simulink model "momentum based estimator"  (R2022a)
settings: Solver=VariableStepAuto  StartTime=0.0  StopTime=30  RelTol=1e-3
values from neighbouring files (symbols this model uses):
  Ib = diag([1.2416 1.2416 2*1.2416])    [momentum based estimator.m]
  k11 = wn1    (= 80)    [momentum based estimator.m]
  k12 = wn2^2/k22    (= 57.1428571429)    [momentum based estimator.m]
  k13 = wn3^3/k33/k23    (= 35.8139534884)    [momentum based estimator.m]
  k14 = wn4^4/k24/k34/k44    (= 33.3333333333)    [momentum based estimator.m]
  k15 = wn5^5/k25/k35/k45/k55    (= 30.2941176471)    [momentum based estimator.m]
  k22 = 1.4*wn2    (= 112)    [momentum based estimator.m]
  k23 = 2.15*wn3^2/k33    (= 94.6)    [momentum based estimator.m]
  k24 = 2.7*wn4^3/k34/k44    (= 71.4705882353)    [momentum based estimator.m]
  k25 = 3.4*wn5^4/k35/k45/k55    (= 63.6727272727)    [momentum based estimator.m]
  k33 = 1.75*wn3    (= 134.75)    [momentum based estimator.m]
  k34 = 3.4*wn4^2/k44    (= 145.714285714)    [momentum based estimator.m]
  k35 = 5.5*wn5^3/k55/k45    (= 113.3)    [momentum based estimator.m]
  k44 = 2.1*wn4    (= 189)    [momentum based estimator.m]
  k45 = 5*wn5^2/k55    (= 183.928571429)    [momentum based estimator.m]
  k55 = 2.8*wn5    (= 288.4)    [momentum based estimator.m]
  mass = 1.1    [momentum based estimator.m]
undefined symbols (not defined in the file or in its folder): DiscIntNeverNeededParam
settings Model: Creator=ThinkPad  LastModifiedBy=ThinkPad

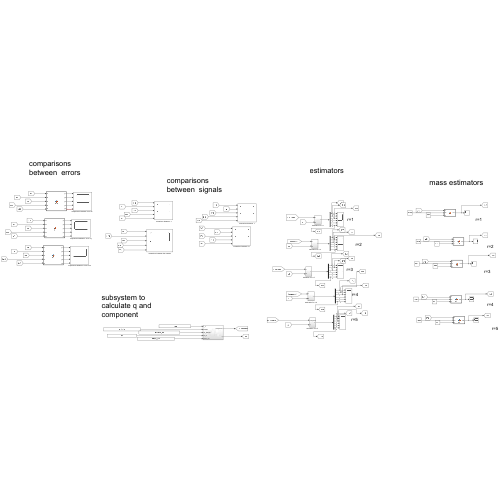
[thumbnail: Simulink's stored preview of the top-level diagram]
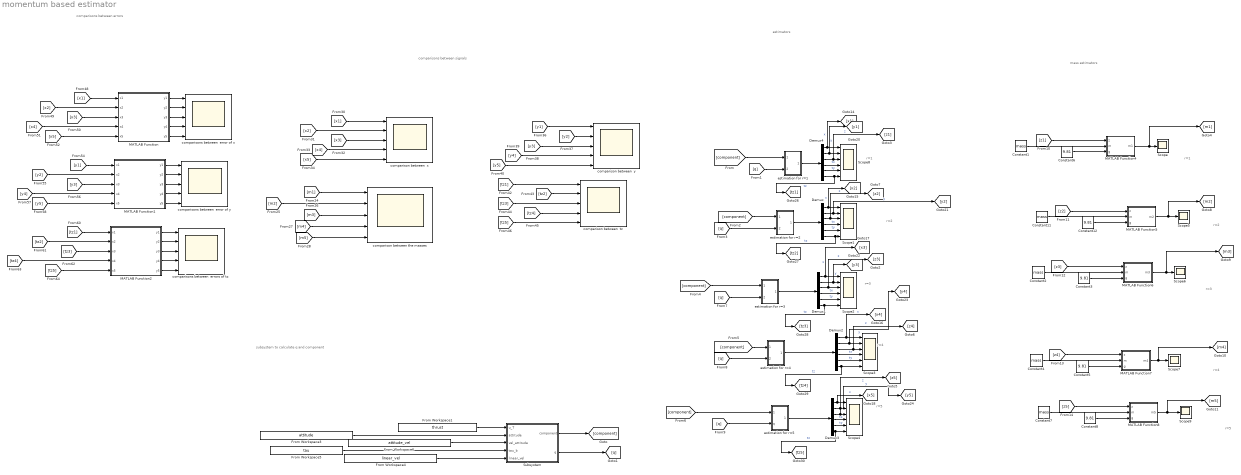
== system momentum based estimator ==
  note: r=1
  note: r=3
  note: r=2
  note: estimators
  note: comparisons between errors
  note: r=5
  note: r=4
  note: comparisons between signals
  note: mass estimators
  note: subsystem to calculate q and component
  note: r=1
  note: r=2
  note: r=3
  note: r=4
  note: r=5
  Constant{1..2,4,7,11} (5 alike) : Constant  Value=mass
  Constant{3,5..6,8,12} (5 alike) : Constant  Value=9.81
  Demux{,1..4} (5 alike) : Demux  Outputs=6
  From Workspace1 : FromWorkspace  VariableName=thrust  SampleTime=0.001
  From Workspace3 : FromWorkspace  VariableName=attitude  SampleTime=0.001
  From Workspace4 : FromWorkspace  VariableName=linear_vel  SampleTime=0.001
  From Workspace5 : FromWorkspace  VariableName=tau  SampleTime=0.001
  From Workspace6 : FromWorkspace  VariableName=attitude_vel  SampleTime=0.001
  MATLAB Function : MATLAB Function  TreatAsAtomicUnit=on
  MATLAB Function1 : MATLAB Function  TreatAsAtomicUnit=on
  MATLAB Function2 : MATLAB Function  TreatAsAtomicUnit=on
  MATLAB Function4 : MATLAB Function  TreatAsAtomicUnit=on
  MATLAB Function5 : MATLAB Function  TreatAsAtomicUnit=on
  MATLAB Function6 : MATLAB Function  TreatAsAtomicUnit=on
  MATLAB Function7 : MATLAB Function  TreatAsAtomicUnit=on
  MATLAB Function8 : MATLAB Function  TreatAsAtomicUnit=on
  Scope{,5..7,9} (5 alike) : Scope
  Scope{1..4,8} (5 alike) : Scope  NumInputPorts=6
  Subsystem : Subsystem
  comparison between  tz : Scope  NumInputPorts=5
  comparison between  x : Scope  NumInputPorts=5
  comparison between  y : Scope  NumInputPorts=5
  comparison between the masses : Scope  NumInputPorts=5
  comparisons between  error of x : Scope  NumInputPorts=5
  comparisons between  error of y : Scope  NumInputPorts=5
  comparisons between  errors of tz : Scope  NumInputPorts=5
  estimation for r=1 : Subsystem
  estimation for r=2 : Subsystem
  estimation for r=3 : Subsystem
  estimation for r=4 : Subsystem
  estimation for r=5 : Subsystem
  wires:
  Demux1/3 -> Scope2/3, [z3]  "z"
  [component] -> estimation for r=4/1(In1)
  Demux2/5 -> Scope3/5  "ty"
  [component] -> estimation for r=1/1(In1)
  Demux/3 -> [z2], Scope1/3  "z"
  estimation for r=2/1(Out1) -> Demux/1
  Demux/5 -> Scope1/5  "ty"
  [m5] -> comparison between the masses/5
  Demux4/6 -> [tz1], Scope8/6  "tz"
  Demux3/6 -> [tz5], Scope4/6  "tz"
  From Workspace3/1 -> Subsystem/2(attitude)
  Demux4/2 -> [y1], Scope8/2  "y"
  From Workspace6/1 -> Subsystem/3(vel_attitude)
  Demux4/3 -> [z1], Scope8/3  "z"
  estimation for r=5/1(Out1) -> Demux3/1
  Demux3/2 -> [y5], Scope4/2  "y"
  estimation for r=4/1(Out1) -> Demux2/1
  Demux/2 -> [y2], Scope1/2  "y"
  From Workspace5/1 -> Subsystem/4(tau_b)
  [x4] -> MATLAB Function/4(x4)
  [x2] -> MATLAB Function/2(x2)
  [q] -> estimation for r=4/2(In2)
  MATLAB Function1/5(y5) -> comparisons between  error of y/5
  [q] -> estimation for r=1/2(In2)
  [m2] -> comparison between the masses/2
  [y5] -> MATLAB Function1/5(x5)
  Subsystem/2(q) -> [q]
  MATLAB Function/2(y2) -> comparisons between  error of x/2
  [y2] -> MATLAB Function1/2(x2)
  [y1] -> MATLAB Function1/1(x1)
  [tz5] -> MATLAB Function2/5(x5)
  MATLAB Function2/5(y5) -> comparisons between  errors of tz/5
  MATLAB Function2/3(y3) -> comparisons between  errors of tz/3
  Demux2/3 -> [z4], Scope3/3  "z"
  From Workspace4/1 -> Subsystem/5(linear_vel)
  MATLAB Function1/3(y3) -> comparisons between  error of y/3
  Demux1/6 -> [tz3], Scope2/6  "tz"
  Demux3/4 -> Scope4/4  "tx"
  Demux2/4 -> Scope3/4  "tx"
  [component] -> estimation for r=3/1(In1)
  estimation for r=1/1(Out1) -> Demux4/1
  Demux3/1 -> [x5], Scope4/1  "x"
  MATLAB Function1/2(y2) -> comparisons between  error of y/2
  [component] -> estimation for r=5/1(component)
  Demux/1 -> [x2], Scope1/1  "x"
  From Workspace1/1 -> Subsystem/1(u_T)
  [tz3] -> comparison between  tz/3
  Demux2/6 -> [tz4], Scope3/6  "tz"
  [tz4] -> comparison between  tz/4
  [x1] -> comparison between  x/1
  Demux/6 -> [tz2], Scope1/6  "tz"
  Demux4/5 -> Scope8/5  "ty"
  Demux1/2 -> [y3], Scope2/2  "y"
  estimation for r=3/1(Out1) -> Demux1/1
  [tz1] -> comparison between  tz/1
  [q] -> estimation for r=5/2(q)
  [x5] -> comparison between  x/5
  [y4] -> comparison between  y/4
  [tz2] -> comparison between  tz/2
  [x4] -> comparison between  x/4
  [x3] -> comparison between  x/3
  [x2] -> comparison between  x/2
  [y1] -> comparison between  y/1
  [y3] -> comparison between  y/3
  [y2] -> comparison between  y/2
  [tz5] -> comparison between  tz/5
  [x3] -> MATLAB Function/3(x3)
  Demux3/3 -> [z5], Scope4/3  "z"
  [m4] -> comparison between the masses/4
  MATLAB Function/3(y3) -> comparisons between  error of x/3
  ? -> ?
  [y3] -> MATLAB Function1/3(x3)
  [y4] -> MATLAB Function1/4(x4)
  MATLAB Function/4(y4) -> comparisons between  error of x/4
  Demux2/2 -> [y4], Scope3/2  "y"
  Demux3/5 -> Scope4/5  "ty"
  [y5] -> comparison between  y/5
  [x5] -> MATLAB Function/5(x5)
  Demux1/5 -> Scope2/5  "ty"
  Demux2/1 -> [x4], Scope3/1  "x"
  [component] -> estimation for r=2/1(In1)
  [q] -> estimation for r=3/2(In2)
  Subsystem/1(component) -> [component]
  [x1] -> MATLAB Function/1(x1)
  Demux4/4 -> Scope8/4  "tx"
  Demux1/1 -> [x3], Scope2/1  "x"
  Demux4/1 -> [x1], Scope8/1  "x"
  [q] -> estimation for r=2/2(In2)
  Demux/4 -> Scope1/4  "tx"
  MATLAB Function/5(y5) -> comparisons between  error of x/5
  MATLAB Function/1(y1) -> comparisons between  error of x/1
  [tz2] -> MATLAB Function2/2(x2)
  Demux1/4 -> Scope2/4  "tx"
  MATLAB Function1/4(y4) -> comparisons between  error of y/4
  [m1] -> comparison between the masses/1
  MATLAB Function2/4(y4) -> comparisons between  errors of tz/4
  [tz4] -> MATLAB Function2/4(x4)
  [tz1] -> MATLAB Function2/1(x1)
  [tz3] -> MATLAB Function2/3(x3)
  MATLAB Function2/2(y2) -> comparisons between  errors of tz/2
  MATLAB Function2/1(y1) -> comparisons between  errors of tz/1
  [m3] -> comparison between the masses/3
  MATLAB Function1/1(y1) -> comparisons between  error of y/1
  [z1] -> MATLAB Function4/1(z)
  Constant1/1 -> MATLAB Function4/2(m)
  Constant6/1 -> MATLAB Function4/3(g)
  [z2] -> MATLAB Function5/1(z)
  Constant11/1 -> MATLAB Function5/2(m)
  Constant12/1 -> MATLAB Function5/3(g)
  MATLAB Function5/1(m2) -> Scope5/1, [m2]
  MATLAB Function6/1(m3) -> Scope6/1, [m3]
  Constant3/1 -> MATLAB Function6/3(g)
  Constant2/1 -> MATLAB Function6/2(m)
  [z3] -> MATLAB Function6/1(z)
  MATLAB Function7/1(m4) -> Scope7/1, [m4]
  Constant5/1 -> MATLAB Function7/3(g)
  Constant4/1 -> MATLAB Function7/2(m)
  [z4] -> MATLAB Function7/1(z)
  MATLAB Function8/1(m5) -> Scope9/1, [m5]
  Constant8/1 -> MATLAB Function8/3(g)
  Constant7/1 -> MATLAB Function8/2(m)
  [z5] -> MATLAB Function8/1(z)
  MATLAB Function4/1(m1) -> [m1], Scope/1

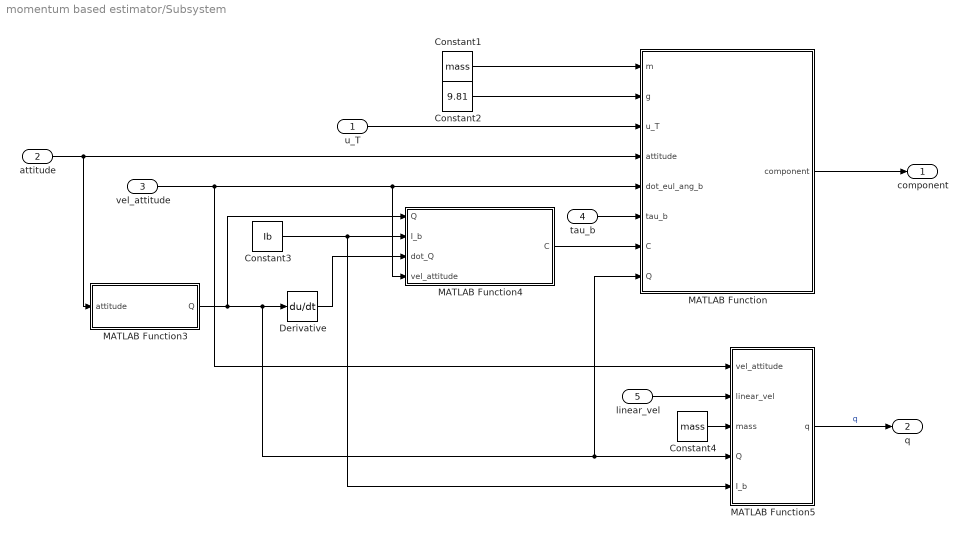
== system momentum based estimator/Subsystem ==
  u_T : Inport
  attitude : Inport  Port=2
  vel_attitude : Inport  Port=3
  tau_b : Inport  Port=4
  linear_vel : Inport  Port=5
  Constant1 : Constant  Value=mass
  Constant2 : Constant  Value=9.81
  Constant3 : Constant  Value=Ib
  Constant4 : Constant  Value=mass
  Derivative : Derivative
  MATLAB Function : MATLAB Function  TreatAsAtomicUnit=on
  MATLAB Function3 : MATLAB Function  TreatAsAtomicUnit=on
  MATLAB Function4 : MATLAB Function  TreatAsAtomicUnit=on
  MATLAB Function5 : MATLAB Function  TreatAsAtomicUnit=on
  component : Outport
  q : Outport  Port=2
  wires:
  Constant4/1 -> MATLAB Function5/3(mass)
  Constant1/1 -> MATLAB Function/1(m)
  MATLAB Function3/1(Q) -> Derivative/1, MATLAB Function5/4(Q), MATLAB Function/8(Q), MATLAB Function4/1(Q)
  Constant2/1 -> MATLAB Function/2(g)
  attitude/1 -> MATLAB Function3/1(attitude), MATLAB Function/4(attitude)
  Derivative/1 -> MATLAB Function4/3(dot_Q)
  Constant3/1 -> MATLAB Function5/5(I_b), MATLAB Function4/2(I_b)
  MATLAB Function4/1(C) -> MATLAB Function/7(C)
  MATLAB Function5/1(q) -> q/1  "q"
  tau_b/1 -> MATLAB Function/6(tau_b)
  u_T/1 -> MATLAB Function/3(u_T)
  MATLAB Function/1(component) -> component/1
  linear_vel/1 -> MATLAB Function5/2(linear_vel)
  vel_attitude/1 -> MATLAB Function5/1(vel_attitude), MATLAB Function4/4(vel_attitude), MATLAB Function/5(dot_eul_ang_b)

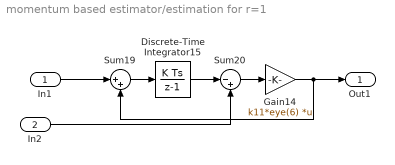
== system momentum based estimator/estimation for r=1 ==
  In1 : Inport
  In2 : Inport  Port=2
  Discrete-Time Integrator15 : DiscreteIntegrator  SampleTime=0.001  ICPrevOutput=DiscIntNeverNeededParam  ICPrevScaledInput=DiscIntNeverNeededParam
  Gain14 : Gain  Gain=k11*eye(6)  Multiplication=Matrix(K*u)
  Sum19 : Sum  Inputs=|++
  Sum20 : Sum  Inputs=|-+
  Out1 : Outport
  wires:
  Gain14/1 -> Out1/1, Sum19/2
  Sum20/1 -> Gain14/1
  In1/1 -> Sum19/1
  Discrete-Time Integrator15/1 -> Sum20/1
  Sum19/1 -> Discrete-Time Integrator15/1
  In2/1 -> Sum20/2

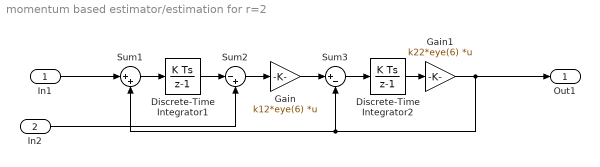
== system momentum based estimator/estimation for r=2 ==
  In1 : Inport
  In2 : Inport  Port=2
  Discrete-Time Integrator1 : DiscreteIntegrator  SampleTime=0.001  ICPrevOutput=DiscIntNeverNeededParam  ICPrevScaledInput=DiscIntNeverNeededParam
  Discrete-Time Integrator2 : DiscreteIntegrator  SampleTime=0.001  ICPrevOutput=DiscIntNeverNeededParam  ICPrevScaledInput=DiscIntNeverNeededParam
  Gain : Gain  Gain=k12*eye(6)  Multiplication=Matrix(K*u)
  Gain1 : Gain  Gain=k22*eye(6)  Multiplication=Matrix(K*u)
  Sum1 : Sum  Inputs=|++
  Sum2 : Sum  Inputs=|-+
  Sum3 : Sum  Inputs=|+-
  Out1 : Outport
  wires:
  Gain1/1 -> Out1/1, Sum1/2, Sum3/2
  Discrete-Time Integrator1/1 -> Sum2/1
  Sum2/1 -> Gain/1
  Sum3/1 -> Discrete-Time Integrator2/1
  Discrete-Time Integrator2/1 -> Gain1/1
  Gain/1 -> Sum3/1
  Sum1/1 -> Discrete-Time Integrator1/1
  In1/1 -> Sum1/1
  In2/1 -> Sum2/2

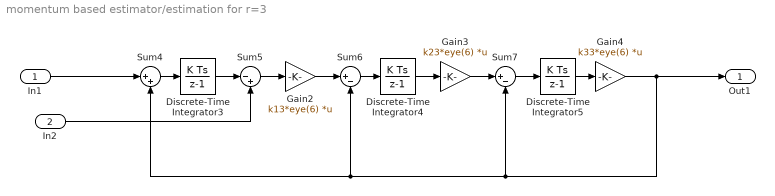
== system momentum based estimator/estimation for r=3 ==
  In1 : Inport
  In2 : Inport  Port=2
  Discrete-Time Integrator3 : DiscreteIntegrator  InitialCondition=0.001  SampleTime=-1  ICPrevOutput=DiscIntNeverNeededParam  ICPrevScaledInput=DiscIntNeverNeededParam
  Discrete-Time Integrator4 : DiscreteIntegrator  SampleTime=0.001  ICPrevOutput=DiscIntNeverNeededParam  ICPrevScaledInput=DiscIntNeverNeededParam
  Discrete-Time Integrator5 : DiscreteIntegrator  SampleTime=0.001  ICPrevOutput=DiscIntNeverNeededParam  ICPrevScaledInput=DiscIntNeverNeededParam
  Gain2 : Gain  Gain=k13*eye(6)  Multiplication=Matrix(K*u)
  Gain3 : Gain  Gain=k23*eye(6)  Multiplication=Matrix(K*u)
  Gain4 : Gain  Gain=k33*eye(6)  Multiplication=Matrix(K*u)
  Sum4 : Sum  Inputs=|++
  Sum5 : Sum  Inputs=|-+
  Sum6 : Sum  Inputs=|+-
  Sum7 : Sum  Inputs=|+-
  Out1 : Outport
  wires:
  Discrete-Time Integrator3/1 -> Sum5/1
  Sum6/1 -> Discrete-Time Integrator4/1
  Gain2/1 -> Sum6/1
  Sum7/1 -> Discrete-Time Integrator5/1
  Sum4/1 -> Discrete-Time Integrator3/1
  Discrete-Time Integrator5/1 -> Gain4/1
  Gain3/1 -> Sum7/1
  Discrete-Time Integrator4/1 -> Gain3/1
  Sum5/1 -> Gain2/1
  Gain4/1 -> Out1/1, Sum4/2, Sum6/2, Sum7/2
  In1/1 -> Sum4/1
  In2/1 -> Sum5/2

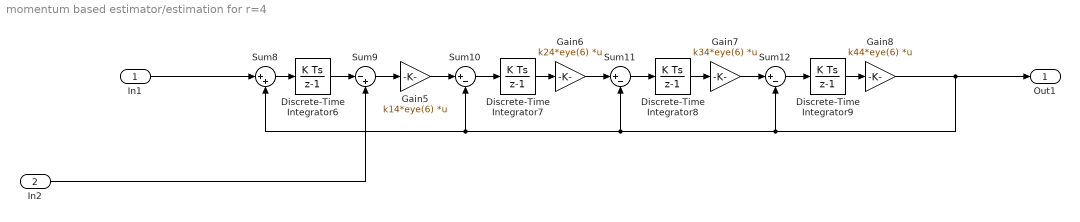
== system momentum based estimator/estimation for r=4 ==
  In1 : Inport
  In2 : Inport  Port=2
  Discrete-Time Integrator{6..9} (4 alike) : DiscreteIntegrator  SampleTime=0.001  ICPrevOutput=DiscIntNeverNeededParam  ICPrevScaledInput=DiscIntNeverNeededParam
  Gain5 : Gain  Gain=k14*eye(6)  Multiplication=Matrix(K*u)
  Gain6 : Gain  Gain=k24*eye(6)  Multiplication=Matrix(K*u)
  Gain7 : Gain  Gain=k34*eye(6)  Multiplication=Matrix(K*u)
  Gain8 : Gain  Gain=k44*eye(6)  Multiplication=Matrix(K*u)
  Sum10 : Sum  Inputs=|+-
  Sum11 : Sum  Inputs=|+-
  Sum12 : Sum  Inputs=|+-
  Sum8 : Sum  Inputs=|++
  Sum9 : Sum  Inputs=|-+
  Out1 : Outport
  wires:
  Gain6/1 -> Sum11/1
  Gain8/1 -> Out1/1, Sum12/2, Sum11/2, Sum8/2, Sum10/2
  Gain5/1 -> Sum10/1
  Discrete-Time Integrator8/1 -> Gain7/1
  Sum8/1 -> Discrete-Time Integrator6/1
  Sum9/1 -> Gain5/1
  Gain7/1 -> Sum12/1
  Discrete-Time Integrator6/1 -> Sum9/1
  Discrete-Time Integrator9/1 -> Gain8/1
  Discrete-Time Integrator7/1 -> Gain6/1
  Sum12/1 -> Discrete-Time Integrator9/1
  Sum11/1 -> Discrete-Time Integrator8/1
  In2/1 -> Sum9/2
  Sum10/1 -> Discrete-Time Integrator7/1
  In1/1 -> Sum8/1

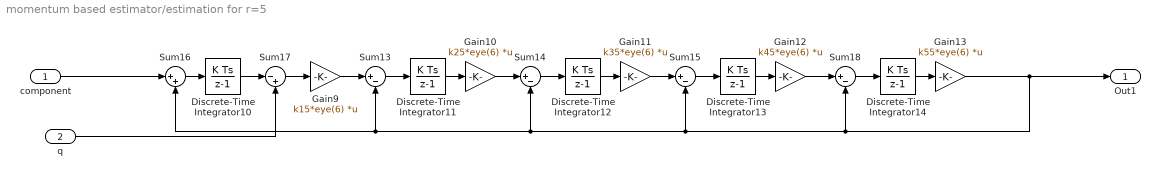
== system momentum based estimator/estimation for r=5 ==
  component : Inport
  q : Inport  Port=2
  Discrete-Time Integrator{10..14} (5 alike) : DiscreteIntegrator  SampleTime=0.001  ICPrevOutput=DiscIntNeverNeededParam  ICPrevScaledInput=DiscIntNeverNeededParam
  Gain10 : Gain  Gain=k25*eye(6)  Multiplication=Matrix(K*u)
  Gain11 : Gain  Gain=k35*eye(6)  Multiplication=Matrix(K*u)
  Gain12 : Gain  Gain=k45*eye(6)  Multiplication=Matrix(K*u)
  Gain13 : Gain  Gain=k55*eye(6)  Multiplication=Matrix(K*u)
  Gain9 : Gain  Gain=k15*eye(6)  Multiplication=Matrix(K*u)
  Sum{13..15,18} (4 alike) : Sum  Inputs=|+-
  Sum16 : Sum  Inputs=|++
  Sum17 : Sum  Inputs=|-+
  Out1 : Outport
  wires:
  Gain9/1 -> Sum13/1
  Sum14/1 -> Discrete-Time Integrator12/1
  Sum15/1 -> Discrete-Time Integrator13/1
  Gain13/1 -> Out1/1, Sum18/2, Sum15/2, Sum14/2, Sum16/2, Sum13/2
  Gain11/1 -> Sum15/1
  Sum18/1 -> Discrete-Time Integrator14/1
  Sum16/1 -> Discrete-Time Integrator10/1
  Discrete-Time Integrator13/1 -> Gain12/1
  Gain12/1 -> Sum18/1
  Discrete-Time Integrator11/1 -> Gain10/1
  Sum17/1 -> Gain9/1
  Discrete-Time Integrator10/1 -> Sum17/1
  Sum13/1 -> Discrete-Time Integrator11/1
  Discrete-Time Integrator12/1 -> Gain11/1
  Discrete-Time Integrator14/1 -> Gain13/1
  Gain10/1 -> Sum14/1
  component/1 -> Sum16/1
  q/1 -> Sum17/2

== matlab function momentum based estimator/Subsystem/MATLAB Function3 ==
  data: attitude input; Q output
function Q = fcn(attitude)
Q=[ 1 0 -sin(attitude(2));
    0 cos(attitude(1)) cos(attitude(2))*sin(attitude(1));
    0 -sin(attitude(1)) cos(attitude(2))*cos(attitude(1))];

== matlab function momentum based estimator/Subsystem/MATLAB Function4 ==
  data: Q input; C output; I_b input; dot_Q input; vel_attitude input
function C = fcn(Q,I_b,dot_Q,vel_attitude)
C=Q'*skew(Q*vel_attitude)*I_b*Q+Q'*I_b*dot_Q;

function S = skew(v)
if(numel(v)~= 1)
S= [0 -v(3) v(2); 
    v(3) 0 -v(1);
    -v(2) v(1) 0];
else
S= zeros(3);
end

== matlab function momentum based estimator/Subsystem/MATLAB Function5 ==
  data: vel_attitude input; linear_vel input; mass input; q output; Q input; I_b input
function q = fcn(vel_attitude,linear_vel,mass,Q,I_b)
M=Q'*I_b*Q;
q=[ mass*eye(3) zeros(3);zeros(3) M]*[linear_vel;vel_attitude];

== matlab function momentum based estimator/MATLAB Function2 ==
  data: y1 output; y2 output; y3 output; y4 output; y5 output; x1 input; x2 input; x3 input; x4 input; x5 input
function [y1,y2,y3,y4,y5] = fcn(x1,x2,x3,x4,x5)

y1=0.1-x1;
y2=0.1-x2;
y3=0.1-x3;
y4=0.1-x4;
y5=0.1-x5;

== matlab function momentum based estimator/MATLAB Function5 ==
  data: z input; m2 output; m input; g input
function m2 = fcn(z,m,g)

m2=m+(z/g);

== matlab function momentum based estimator/MATLAB Function4 ==
  data: z input; m1 output; m input; g input
function m1 = fcn(z,m,g)

m1=m+(z/g);

== matlab function momentum based estimator/Subsystem/MATLAB Function ==
  data: m input; component output; g input; u_T input; attitude input; dot_eul_ang_b input; tau_b input; C input; Q input
function component = fcn(m,g,u_T,attitude,dot_eul_ang_b,tau_b,C,Q)
R_b=eul2rotm([attitude(1) attitude(2) attitude(3)],'XYZ');
component=[  m*g*[0 0 1]'-u_T*R_b*[0 0 1]';
        C'*dot_eul_ang_b+Q'*tau_b];

== matlab function momentum based estimator/MATLAB Function6 ==
  data: z input; m3 output; m input; g input
function m3 = fcn(z,m,g)

m3=m+(z/g);

== matlab function momentum based estimator/MATLAB Function7 ==
  data: z input; m4 output; m input; g input
function m4 = fcn(z,m,g)

m4=m+(z/g);

== matlab function momentum based estimator/MATLAB Function8 ==
  data: z input; m5 output; m input; g input
function m5 = fcn(z,m,g)

m5=m+(z/g);

== matlab function momentum based estimator/MATLAB Function ==
  data: y1 output; y2 output; y3 output; y4 output; y5 output; x1 input; x2 input; x3 input; x4 input; x5 input
function [y1,y2,y3,y4,y5] = fcn(x1,x2,x3,x4,x5)

y1=1-x1;
y2=1-x2;
y3=1-x3;
y4=1-x4;
y5=1-x5;

== matlab function momentum based estimator/MATLAB Function1 ==
  data: y1 output; y2 output; y3 output; y4 output; y5 output; x1 input; x2 input; x3 input; x4 input; x5 input
function [y1,y2,y3,y4,y5] = fcn(x1,x2,x3,x4,x5)

y1=1-x1;
y2=1-x2;
y3=1-x3;
y4=1-x4;
y5=1-x5;
